simulink model "LICENTA_2024"  (R2018b)
settings: Solver=FixedStepDiscrete  StartTime=0.0  StopTime=Inf  RelTol=1e-3  EnableMultiTasking=on
values from neighbouring files (symbols this model uses):
  A = -Rs/Ld    (= -2.40983606557)    [licentam18.m]
  const_cuplu = 0.035    [licentam18.m]
  factor_conversie = (1/Rshunt)*(1/10)*(vref/4095)    (= 0.0115122972266)    [licentam18.m]
  FED = uint16(50)    [licentam18.m]
  MaxIter_1_ms_eCAP_wait = MinDetectSpeed_period/T_pos    (= 375)    [licentam18.m]
  pp = 16/2    (= 8)    [licentam18.m]
  RED = uint16(50)    [licentam18.m]
  T_pos = 0.0005    [licentam18.m]
  TBPRD1 = uint16(TPWM/(2*TTBCLK))    [licentam18.m]
  Tf = 0.015    [licentam18.m]
  Tf_spd = 0.01    [licentam18.m]
  Ts = Ts_crt_control    (= 3.33333333333e-05)    [licentam18.m]
  TTBCLK = 1/F    (= 5e-09)    [licentam18.m]
undefined symbols (not defined in the file or in its folder): Down, GPTRIP1SEL, GPTRIP2SEL, K, offset_ADC, radians, TZ1, TZ2, Up
libraries: tiiqmathlib x39, c2802xlib x9, c2837xDlib x6, simulink x5, c280xlib x4, c28xdmclib x2, c2000lib x1
(part 1 of 2)
settings Model: ExtModeTrigDuration=8  Creator=mocan  LastModifiedBy=mocan
settings SolverCC: AutoInsertRateTranBlk=on
settings OptimizationCC: DefaultUnderspecifiedDataType=single  EnhancedBackFolding=on  PassReuseOutputArgsAs=Individual arguments  MaxStackSize=512  OptimizeBlockOrder=speed  DifferentSizesBufferReuse=on  OptimizationCustomize=off
settings DebuggingCC: ParameterPrecisionLossMsg=none  ParameterTunabilityLossMsg=error
settings HardwareCC: ProdBitPerChar=16  ProdBitPerInt=16  ProdBitPerPointer=32  ProdBitPerSizeT=32  ProdBitPerPtrDiffT=32  ProdLargestAtomicInteger=Integer  ProdLargestAtomicFloat=None  ProdWordSize=16  ProdLongLongMode=on  ProdHWDeviceType=Texas Instruments->C2000
settings SFSimCC: MATLABDynamicMemAlloc=off
settings RTWCC: SystemTargetFile=ert.tlc  HardwareBoard=TI Delfino F28379D LaunchPad  TemplateMakefile=ert_default_tmf  GenerateReport=on  Toolchain=Texas Instruments Code Composer Studio (C2000)  IncludeHyperlinkInReport=on  LaunchReport=on  GenerateTraceInfo=on  GenerateTraceReport=on  GenerateTraceReportSl=on  GenerateTraceReportSf=on  GenerateTraceReportEml=on
settings CodeAppCC: ForceParamTrailComments=on  IgnoreCustomStorageClasses=off  OperatorAnnotations=on  SimulinkDataObjDesc=on  SFDataObjDesc=on  InsertBlockDesc=on
settings ERTTargetCC: CodeReplacementLibrary=TI C28x

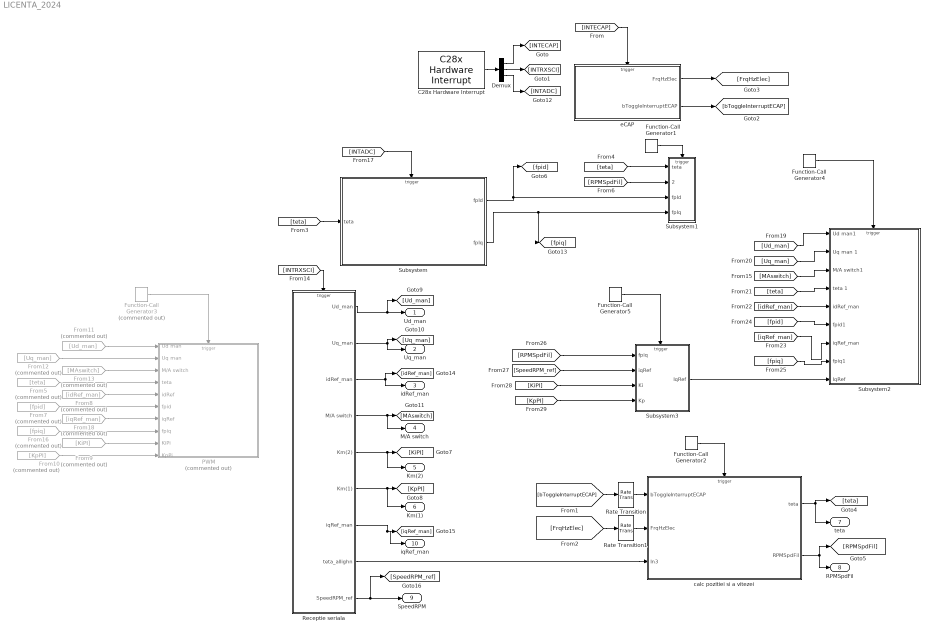
== system LICENTA_2024 ==
  C28x Hardware Interrupt : c2000lib/Scheduling/C28x Hardware Interrupt  irqnumbers=[4,9,1]  pienumbers=[1,1,1]  irqpriorities=[1, 1, 1]  irqpreempts=[0 0 0]  showinput=off  dspchiptype=C280X
      settings: SourceProductBaseCode=TIC2000
  Demux : Demux  Outputs=3
  From10 : From  Commented=on  GotoTag=KpPI
  From11 : From  Commented=on  GotoTag=Ud_man
  From12 : From  Commented=on  GotoTag=Uq_man
  From13 : From  Commented=on  GotoTag=MAswitch
  From16 : From  Commented=on  GotoTag=fpiq
  From18 : From  Commented=on  GotoTag=iqRef_man
  From5 : From  Commented=on  GotoTag=teta
  From7 : From  Commented=on  GotoTag=fpid
  From8 : From  Commented=on  GotoTag=idRef_man
  From9 : From  Commented=on  GotoTag=KiPI
  Function-Call Generator1 : simulink/Ports & Subsystems/Function-Call Generator  sample_time=0.03  numberOfIterations=1
  Function-Call Generator2 : simulink/Ports & Subsystems/Function-Call Generator  sample_time=T_pos  numberOfIterations=1
  Function-Call Generator3 : simulink/Ports & Subsystems/Function-Call Generator  Commented=on  sample_time=Ts_crt_control  numberOfIterations=1
  Function-Call Generator4 : simulink/Ports & Subsystems/Function-Call Generator  sample_time=Ts_crt_control  numberOfIterations=1
  Function-Call Generator5 : simulink/Ports & Subsystems/Function-Call Generator  sample_time=T_pos  numberOfIterations=1
  PWM : Subsystem  Commented=on
  Rate Transition : RateTransition  Integrity=off  OutPortSampleTime=T_pos
  Rate Transition1 : RateTransition  Integrity=off  OutPortSampleTime=T_pos
  "Receptie seriala " : Subsystem
  Subsystem : Subsystem
  Subsystem1 : Subsystem
  Subsystem2 : Subsystem
  Subsystem3 : Subsystem
  calc pozitiei si a vitezei : Subsystem
  eCAP : Subsystem
  Ud_man : Outport  VectorParamsAs1DForOutWhenUnconnected=on
  Uq_man : Outport  Port=2  VectorParamsAs1DForOutWhenUnconnected=on
  idRef_man : Outport  Port=3  VectorParamsAs1DForOutWhenUnconnected=on
  M/A switch : Outport  Port=4  VectorParamsAs1DForOutWhenUnconnected=on
  Km(2) : Outport  Port=5  VectorParamsAs1DForOutWhenUnconnected=on
  Km(1) : Outport  Port=6  VectorParamsAs1DForOutWhenUnconnected=on
  teta : Outport  Port=7  VectorParamsAs1DForOutWhenUnconnected=on
  RPMSpdFil : Outport  Port=8  VectorParamsAs1DForOutWhenUnconnected=on
  SpeedRPM : Outport  Port=9
  iqRef_man : Outport  Port=10
  wires:
  Rate Transition1/1 -> calc pozitiei si a vitezei/2(FrqHzElec)
  [FrqHzElec] -> Rate Transition1/1
  Rate Transition/1 -> calc pozitiei si a vitezei/1(bToggleInterruptECAP)
  [bToggleInterruptECAP] -> Rate Transition/1
  [INTECAP] -> eCAP/Trigger
  eCAP/1(FrqHzElec) -> [FrqHzElec]
  eCAP/2(bToggleInterruptECAP) -> [bToggleInterruptECAP]
  Demux/2 -> [INTRXSCI]
  Demux/1 -> [INTECAP]
  Function-Call Generator2/1 -> calc pozitiei si a vitezei/Trigger
  calc pozitiei si a vitezei/2(RPMSpdFil) -> [RPMSpdFil], RPMSpdFil/1
  Function-Call Generator1/1 -> Subsystem1/Trigger
  calc pozitiei si a vitezei/1(teta) -> [teta], teta/1
  [INTRXSCI] -> "Receptie seriala "/Trigger
  C28x Hardware Interrupt/1 -> Demux/1
  "Receptie seriala "/1(Ud_man) -> [Ud_man], Ud_man/1
  "Receptie seriala "/2(Uq_man) -> Uq_man/1, [Uq_man]
  "Receptie seriala "/4(M/A switch) -> M/A switch/1, [MAswitch]
  "Receptie seriala "/5(Km(2)) -> [KiPI], Km(2)/1
  "Receptie seriala "/6(Km(1)) -> Km(1)/1, [KpPI]
  Function-Call Generator3/1 -> PWM/Trigger
  Demux/3 -> [INTADC]
  [INTADC] -> Subsystem/Trigger
  [teta] -> Subsystem/1(teta)
  Subsystem/1(fpId) -> [fpid], Subsystem1/3(fpId)
  "Receptie seriala "/7(iqRef_man) -> iqRef_man/1, [iqRef_man]
  "Receptie seriala "/3(idRef_man) -> idRef_man/1, [idRef_man]
  From11/1 -> PWM/1(Ud man)
  From12/1 -> PWM/2("Uq man ")
  From13/1 -> PWM/3(M/A switch)
  From5/1 -> PWM/4("teta ")
  From8/1 -> PWM/5(idRef)
  From7/1 -> PWM/6(fpid)
  From16/1 -> PWM/8(fpiq)
  From18/1 -> PWM/7(iqRef)
  From9/1 -> PWM/9(KiPi)
  From10/1 -> PWM/10(KpPi)
  "Receptie seriala "/8(teta_allighn) -> calc pozitiei si a vitezei/3(In3)
  Function-Call Generator4/1 -> Subsystem2/Trigger
  [MAswitch] -> Subsystem2/3(M/A switch1)
  [Ud_man] -> Subsystem2/1(Ud man1)
  [teta] -> Subsystem2/4(teta 1)
  [idRef_man] -> Subsystem2/5(idRef_man)
  [iqRef_man] -> Subsystem2/7(iqRef_man)
  [fpid] -> Subsystem2/6(fpid1)
  [fpiq] -> Subsystem2/8(fpiq1)
  "Receptie seriala "/9(SpeedRPM_ref) -> SpeedRPM/1, [SpeedRPM_ref]
  [RPMSpdFil] -> Subsystem3/1(fpiq)
  [SpeedRPM_ref] -> Subsystem3/2(iqRef)
  Function-Call Generator5/1 -> Subsystem3/Trigger
  [Uq_man] -> Subsystem2/2(Uq man 1)
  Subsystem3/1(IqRef) -> Subsystem2/9(IqRef)
  Subsystem/2(fpIq) -> [fpiq], Subsystem1/4(fpIq)
  [teta] -> Subsystem1/1("teta ")
  [RPMSpdFil] -> Subsystem1/2("RPMSpdFil ")
  [KiPI] -> Subsystem3/3(Ki)
  [KpPI] -> Subsystem3/4(Kp)

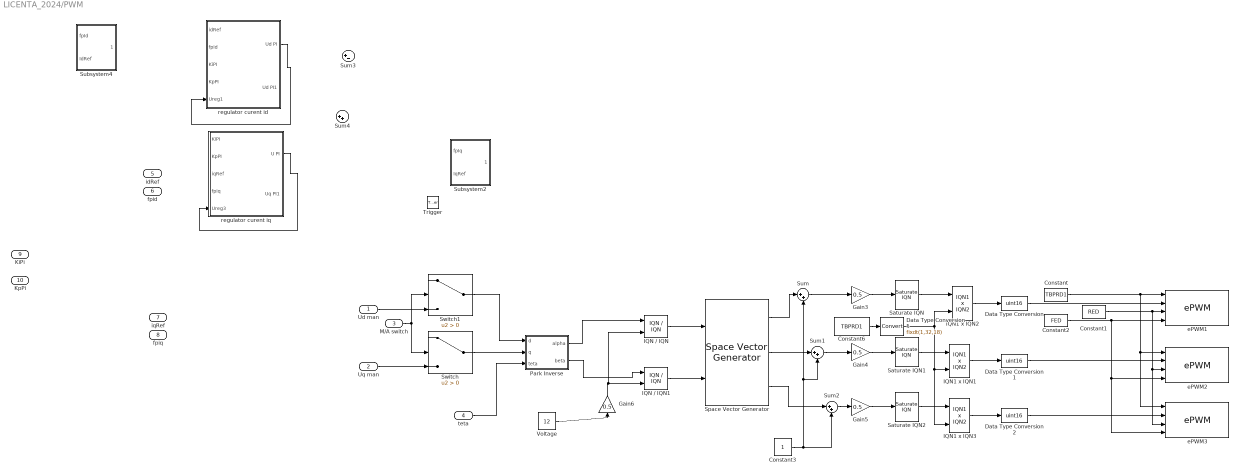
== system LICENTA_2024/PWM ==
  Ud man : Inport
  "Uq man " : Inport  Port=2
  M/A switch : Inport  Port=3
  "teta " : Inport  Port=4
  idRef : Inport  Port=5
  fpid : Inport  Port=6
  iqRef : Inport  Port=7
  fpiq : Inport  Port=8
  KiPi : Inport  Port=9
  KpPi : Inport  Port=10
  Trigger : TriggerPort  TriggerType=function-call  VariantControl=Variant  PortDimensions=1
  Constant : Constant  Value=TBPRD1
  Constant1 : Constant  Value=RED
  Constant2 : Constant  Value=FED
  Constant3 : Constant  OutDataTypeStr=fixdt(1,32,24)
  Constant6 : Constant  Value=TBPRD1
  Data Type Conversion : DataTypeConversion  OutDataTypeStr=uint16
  Data Type Conversion1 : DataTypeConversion  OutDataTypeStr=uint16
  Data Type Conversion2 : DataTypeConversion  OutDataTypeStr=uint16
  Data Type Conversion5 : DataTypeConversion  OutDataTypeStr=fixdt(1,32,18)
  Gain{3..6} (4 alike) : Gain  Gain=0.5  OutDataTypeStr=Inherit: Same as input
  IQN / IQN : tiiqmathlib/IQN // IQN
      settings: SourceProductName=Embedded Coder Support Package for Texas Instruments C2000 Processors  SourceProductBaseCode=TIC2000
  IQN / IQN1 : tiiqmathlib/IQN // IQN
      settings: SourceProductName=Embedded Coder Support Package for Texas Instruments C2000 Processors  SourceProductBaseCode=TIC2000
  IQN1 x IQN1 : tiiqmathlib/IQN1 x IQN2  Q=10
      settings: SourceProductName=Embedded Coder Support Package for Texas Instruments C2000 Processors  SourceProductBaseCode=TIC2000
  IQN1 x IQN2 : tiiqmathlib/IQN1 x IQN2  Q=10
      settings: SourceProductName=Embedded Coder Support Package for Texas Instruments C2000 Processors  SourceProductBaseCode=TIC2000
  IQN1 x IQN3 : tiiqmathlib/IQN1 x IQN2  Q=10
      settings: SourceProductName=Embedded Coder Support Package for Texas Instruments C2000 Processors  SourceProductBaseCode=TIC2000
  Park Inverse : Subsystem
  Saturate IQN : tiiqmathlib/Saturate IQN  pos=0.95  neg=0.05
      settings: SourceProductName=Embedded Coder Support Package for Texas Instruments C2000 Processors  SourceProductBaseCode=TIC2000
  Saturate IQN1 : tiiqmathlib/Saturate IQN  pos=0.95  neg=0.05
      settings: SourceProductName=Embedded Coder Support Package for Texas Instruments C2000 Processors  SourceProductBaseCode=TIC2000
  Saturate IQN2 : tiiqmathlib/Saturate IQN  pos=0.95  neg=0.05
      settings: SourceProductName=Embedded Coder Support Package for Texas Instruments C2000 Processors  SourceProductBaseCode=TIC2000
  Space Vector Generator : c28xdmclib/Space Vector Generator
      settings: SourceProductName=Embedded Coder Support Package for Texas Instruments C2000 Processors  SourceProductBaseCode=TIC2000
  Subsystem2 : Subsystem
  Subsystem4 : Subsystem
  Sum{,1..2,4} (4 alike) : Sum  Inputs=|++
  Sum3 : Sum  Inputs=|+-
  Switch : Switch  Criteria=u2 > Threshold
  Switch1 : Switch  Criteria=u2 > Threshold
  "Voltage " : Constant  Value=12  OutDataTypeStr=fixdt(1,32,20)
  ePWM1 : c2802xlib/ePWM  useModule=ePWM1  ePWMxLINKTBPRD=Not Linked  periodUnits=Clock cycles  timerSource=Input port  timerPeriod_clk=TBPRD1+1  timerPeriod_sec=0.0001  tbshadow=Counter equals to zero  countingMode=Up-Down  phaseActiveEnable=Disable  phaseDirection=Count up after sync  phaseActive=0  synchronizationEnable=off  dcaevt1Sync=off  dcbevt1Sync=off  synchronizationOption=Counter equals to zero (CTR=Zero)  clockPrescale=1  HSclockPrescale=1  enswap=off  ePWMxAStatus=on  ePWMxAactionLogic1=Do nothing  ePWMxAactionLogic2=Do nothing  ePWMxAactionLogic3=Clear  ePWMxAactionLogic4=Set  ePWMxAactionLogic5=Do nothing  ePWMxAactionLogic6=Do nothing  ePWMxALoadMode=Load on counter equals to zero (CTR=Zero)  ePWMxACSFenable=off  ePWMxACSFvalue=Forcing disable  ePWMxASFreload=Zero  ePWMxBStatus=off  ePWMxBactionLogic1=Set  ePWMxBactionLogic2=Clear  ePWMxBactionLogic3=Do nothing  ePWMxBactionLogic4=Do nothing  ePWMxBactionLogic5=Clear  ePWMxBactionLogic6=Set  ePWMxBLoadMode=Load on counter equals to zero (CTR=Zero)  ePWMxBCSFenable=off  ePWMxBCSFvalue=Forcing disable  ePWMxBSFreload=Zero  ePWNxBOutWay=off  ePWMxLINKCMPA=Not Linked  CMPAUnits=Clock cycles  CMPASource=Input port  CMPAValue_per=50  CMPAValue_clk=0  enCMPAshadow=Counter equals to zero  ePWMxLINKCMPB=Not Linked  CMPBUnits=Clock cycles  CMPBSource=Specify via dialog  CMPBValue_per=50  CMPBValue_clk=0  enCMPBshadow=Counter equals to zero  ePWMxLINKCMPC=Not Linked  CMPCUnits=Clock cycles  CMPCSource=Specify via dialog  CMPCValue_per=50  CMPCValue_clk=32000  enCMPCshadow=Counter equals to zero  ePWMxLINKCMPD=Not Linked  CMPDUnits=Clock cycles  CMPDSource=Specify via dialog  CMPDValue_per=50  CMPDValue_clk=32000  enCMPDshadow=Counter equals to zero  enableDBePWMxA=on  enableDBePWMxB=on  enhalfcycle=off  DBpolarity=Active high complementary (AHC)  DBedgeDelay=Positive  DBSource_ePWMxA=ePWMxA  DBSource_ePWMxB=ePWMxA  DBperiodSource=Input port  REDperiod=0  FEDperiod=0  adcstartModuleA=on  adcrequestEventA=First event  adcstartEventA=Digital Compare Module A Event 1 start of conversion (DCAEVT1.soc)  adcstartEventA_type2=Counter equals to period (CTR=PRD)  adcstartModuleB=off  adcrequestEventB=First event  adcstartEventB=Counter equals to zero (CTR=Zero)  adcstartEventB_type2=Counter equals to zero (CTR=Zero)  intEn=off  intPrd=First event  intSel=Counter equals to zero (CTR=Zero)  intSel_type2=Counter equals to zero (CTR=Zero)  hrpe=off  enHRPWM=off  HRPWM_LoadMode=Counter equals to period (CTR=PRD)  HRPWM_CTLMode=Duty or Period control mode  HRPWM_EDGMode=Both edge  hrpeb=off  enHRPWMB=off  HRPWM_LoadModeB=Counter equals to zero (CTR=ZERO)  HRPWM_CTLModeB=Duty or Period control mode  HRPWM_EDGModeB=Both edge  enSFO=on  enautoconv=on  chopperEnable=off  chopperFrequency=1  chopperFirstwidth=1  chopperDuty=12.5%  tripZonesource=Specify via dialog  tzselOSHT1=off  tzselOSHT2=off  tzselOSHT3=off  tzselOSHDCAEV1=off  tzselOSHDCBEV1=off  tzselCBC1=off  tzselCBC2=off  tzselCBC3=off  tzselCBCDCAEV2=off  tzselCBCDCBEV2=off  tzselOSHT4=off  tzselOSHT5=off  tzselOSHT6=off  tzselCBC4=off  tzselCBC5=off  tzselCBC6=off  enTzOstIntr=off  enTzCbcIntr=off  enTzDCAEVT1Intr=off  enTzDCAEVT2Intr=off  enTzDCBEVT1Intr=off  enTzDCBEVT2Intr=off  ePWMxAforced=No action  ePWMxBforced=No action  DCAEVT1forced=No action  DCBEVT1forced=No action  DCAEVT2forced=No action  DCBEVT2forced=No action  dcah=Trip Zone 1 input (TZ1)  dcal=Trip Zone 2 input (TZ2)  dcbh=Trip Zone 1 input (TZ1)  dcbl=Trip Zone 2 input (TZ2)  dcah_type2=GPTRIP1SEL/(TZ1)  dcal_type2=GPTRIP2SEL/(TZ2)  dcbh_type2=GPTRIP1SEL/(TZ1)  dcbl_type2=GPTRIP2SEL/(TZ2)  gendcaevt1=Event disabled  gendcaevt2=Event disabled  gendcbevt1=Event disabled  gendcbevt2=Event disabled  dcaevt1src=DCAEVT1 with sync  dcaevt2src=DCAEVT2 with sync  dcbevt1src=DCBEVT1 with sync  dcbevt2src=DCBEVT2 with sync  pulsesel=Counter equals to zero (CTR=Zero)  blankinv=off  blankoffset=0  blankwidth=0  evsrcsel=Filtered version of DCAEVT1 (DCAEVT1FILT)  encape=off  PwmType=C2000_Type4
      settings: SourceProductName=Embedded Coder Support Package for Texas Instruments C2000 Processors
  ePWM2 : c2802xlib/ePWM  useModule=ePWM2  ePWMxLINKTBPRD=Not Linked  periodUnits=Clock cycles  timerSource=Input port  timerPeriod_clk=TBPRD1+1  timerPeriod_sec=0.0001  tbshadow=Counter equals to zero  countingMode=Up-Down  phaseActiveEnable=Disable  phaseDirection=Count up after sync  phaseActive=0  synchronizationEnable=off  dcaevt1Sync=off  dcbevt1Sync=off  synchronizationOption=Counter equals to zero (CTR=Zero)  clockPrescale=1  HSclockPrescale=1  enswap=off  ePWMxAStatus=on  ePWMxAactionLogic1=Do nothing  ePWMxAactionLogic2=Do nothing  ePWMxAactionLogic3=Clear  ePWMxAactionLogic4=Set  ePWMxAactionLogic5=Do nothing  ePWMxAactionLogic6=Do nothing  ePWMxALoadMode=Load on counter equals to zero (CTR=Zero)  ePWMxACSFenable=off  ePWMxACSFvalue=Forcing disable  ePWMxASFreload=Zero  ePWMxBStatus=off  ePWMxBactionLogic1=Set  ePWMxBactionLogic2=Clear  ePWMxBactionLogic3=Do nothing  ePWMxBactionLogic4=Do nothing  ePWMxBactionLogic5=Clear  ePWMxBactionLogic6=Set  ePWMxBLoadMode=Load on counter equals to zero (CTR=Zero)  ePWMxBCSFenable=off  ePWMxBCSFvalue=Forcing disable  ePWMxBSFreload=Zero  ePWNxBOutWay=off  ePWMxLINKCMPA=Not Linked  CMPAUnits=Clock cycles  CMPASource=Input port  CMPAValue_per=50  CMPAValue_clk=0  enCMPAshadow=Counter equals to zero  ePWMxLINKCMPB=Not Linked  CMPBUnits=Clock cycles  CMPBSource=Specify via dialog  CMPBValue_per=50  CMPBValue_clk=0  enCMPBshadow=Counter equals to zero  ePWMxLINKCMPC=Not Linked  CMPCUnits=Clock cycles  CMPCSource=Specify via dialog  CMPCValue_per=50  CMPCValue_clk=32000  enCMPCshadow=Counter equals to zero  ePWMxLINKCMPD=Not Linked  CMPDUnits=Clock cycles  CMPDSource=Specify via dialog  CMPDValue_per=50  CMPDValue_clk=32000  enCMPDshadow=Counter equals to zero  enableDBePWMxA=on  enableDBePWMxB=on  enhalfcycle=off  DBpolarity=Active high complementary (AHC)  DBedgeDelay=Positive  DBSource_ePWMxA=ePWMxA  DBSource_ePWMxB=ePWMxA  DBperiodSource=Input port  REDperiod=0  FEDperiod=0  adcstartModuleA=on  adcrequestEventA=First event  adcstartEventA=Digital Compare Module A Event 1 start of conversion (DCAEVT1.soc)  adcstartEventA_type2=Counter equals to period (CTR=PRD)  adcstartModuleB=off  adcrequestEventB=First event  adcstartEventB=Counter equals to zero (CTR=Zero)  adcstartEventB_type2=Counter equals to zero (CTR=Zero)  intEn=off  intPrd=First event  intSel=Counter equals to zero (CTR=Zero)  intSel_type2=Counter equals to zero (CTR=Zero)  hrpe=off  enHRPWM=off  HRPWM_LoadMode=Counter equals to period (CTR=PRD)  HRPWM_CTLMode=Duty or Period control mode  HRPWM_EDGMode=Both edge  hrpeb=off  enHRPWMB=off  HRPWM_LoadModeB=Counter equals to zero (CTR=ZERO)  HRPWM_CTLModeB=Duty or Period control mode  HRPWM_EDGModeB=Both edge  enSFO=on  enautoconv=on  chopperEnable=off  chopperFrequency=1  chopperFirstwidth=1  chopperDuty=12.5%  tripZonesource=Specify via dialog  tzselOSHT1=off  tzselOSHT2=off  tzselOSHT3=off  tzselOSHDCAEV1=off  tzselOSHDCBEV1=off  tzselCBC1=off  tzselCBC2=off  tzselCBC3=off  tzselCBCDCAEV2=off  tzselCBCDCBEV2=off  tzselOSHT4=off  tzselOSHT5=off  tzselOSHT6=off  tzselCBC4=off  tzselCBC5=off  tzselCBC6=off  enTzOstIntr=off  enTzCbcIntr=off  enTzDCAEVT1Intr=off  enTzDCAEVT2Intr=off  enTzDCBEVT1Intr=off  enTzDCBEVT2Intr=off  ePWMxAforced=No action  ePWMxBforced=No action  DCAEVT1forced=No action  DCBEVT1forced=No action  DCAEVT2forced=No action  DCBEVT2forced=No action  dcah=Trip Zone 1 input (TZ1)  dcal=Trip Zone 2 input (TZ2)  dcbh=Trip Zone 1 input (TZ1)  dcbl=Trip Zone 2 input (TZ2)  dcah_type2=GPTRIP1SEL/(TZ1)  dcal_type2=GPTRIP2SEL/(TZ2)  dcbh_type2=GPTRIP1SEL/(TZ1)  dcbl_type2=GPTRIP2SEL/(TZ2)  gendcaevt1=Event disabled  gendcaevt2=Event disabled  gendcbevt1=Event disabled  gendcbevt2=Event disabled  dcaevt1src=DCAEVT1 with sync  dcaevt2src=DCAEVT2 with sync  dcbevt1src=DCBEVT1 with sync  dcbevt2src=DCBEVT2 with sync  pulsesel=Counter equals to zero (CTR=Zero)  blankinv=off  blankoffset=0  blankwidth=0  evsrcsel=Filtered version of DCAEVT1 (DCAEVT1FILT)  encape=off  PwmType=C2000_Type4
      settings: SourceProductName=Embedded Coder Support Package for Texas Instruments C2000 Processors
  ePWM3 : c2802xlib/ePWM  useModule=ePWM3  ePWMxLINKTBPRD=Not Linked  periodUnits=Clock cycles  timerSource=Input port  timerPeriod_clk=TBPRD1+1  timerPeriod_sec=0.0001  tbshadow=Counter equals to zero  countingMode=Up-Down  phaseActiveEnable=Disable  phaseDirection=Count up after sync  phaseActive=0  synchronizationEnable=off  dcaevt1Sync=off  dcbevt1Sync=off  synchronizationOption=Counter equals to zero (CTR=Zero)  clockPrescale=1  HSclockPrescale=1  enswap=off  ePWMxAStatus=on  ePWMxAactionLogic1=Do nothing  ePWMxAactionLogic2=Do nothing  ePWMxAactionLogic3=Clear  ePWMxAactionLogic4=Set  ePWMxAactionLogic5=Do nothing  ePWMxAactionLogic6=Do nothing  ePWMxALoadMode=Load on counter equals to zero (CTR=Zero)  ePWMxACSFenable=off  ePWMxACSFvalue=Forcing disable  ePWMxASFreload=Zero  ePWMxBStatus=off  ePWMxBactionLogic1=Set  ePWMxBactionLogic2=Clear  ePWMxBactionLogic3=Do nothing  ePWMxBactionLogic4=Do nothing  ePWMxBactionLogic5=Clear  ePWMxBactionLogic6=Set  ePWMxBLoadMode=Load on counter equals to zero (CTR=Zero)  ePWMxBCSFenable=off  ePWMxBCSFvalue=Forcing disable  ePWMxBSFreload=Zero  ePWNxBOutWay=off  ePWMxLINKCMPA=Not Linked  CMPAUnits=Clock cycles  CMPASource=Input port  CMPAValue_per=50  CMPAValue_clk=0  enCMPAshadow=Counter equals to zero  ePWMxLINKCMPB=Not Linked  CMPBUnits=Clock cycles  CMPBSource=Specify via dialog  CMPBValue_per=50  CMPBValue_clk=0  enCMPBshadow=Counter equals to zero  ePWMxLINKCMPC=Not Linked  CMPCUnits=Clock cycles  CMPCSource=Specify via dialog  CMPCValue_per=50  CMPCValue_clk=32000  enCMPCshadow=Counter equals to zero  ePWMxLINKCMPD=Not Linked  CMPDUnits=Clock cycles  CMPDSource=Specify via dialog  CMPDValue_per=50  CMPDValue_clk=32000  enCMPDshadow=Counter equals to zero  enableDBePWMxA=on  enableDBePWMxB=on  enhalfcycle=off  DBpolarity=Active high complementary (AHC)  DBedgeDelay=Positive  DBSource_ePWMxA=ePWMxA  DBSource_ePWMxB=ePWMxA  DBperiodSource=Input port  REDperiod=0  FEDperiod=0  adcstartModuleA=on  adcrequestEventA=First event  adcstartEventA=Digital Compare Module A Event 1 start of conversion (DCAEVT1.soc)  adcstartEventA_type2=Counter equals to period (CTR=PRD)  adcstartModuleB=off  adcrequestEventB=First event  adcstartEventB=Counter equals to zero (CTR=Zero)  adcstartEventB_type2=Counter equals to zero (CTR=Zero)  intEn=off  intPrd=First event  intSel=Counter equals to zero (CTR=Zero)  intSel_type2=Counter equals to zero (CTR=Zero)  hrpe=off  enHRPWM=off  HRPWM_LoadMode=Counter equals to period (CTR=PRD)  HRPWM_CTLMode=Duty or Period control mode  HRPWM_EDGMode=Both edge  hrpeb=off  enHRPWMB=off  HRPWM_LoadModeB=Counter equals to zero (CTR=ZERO)  HRPWM_CTLModeB=Duty or Period control mode  HRPWM_EDGModeB=Both edge  enSFO=on  enautoconv=on  chopperEnable=off  chopperFrequency=1  chopperFirstwidth=1  chopperDuty=12.5%  tripZonesource=Specify via dialog  tzselOSHT1=off  tzselOSHT2=off  tzselOSHT3=off  tzselOSHDCAEV1=off  tzselOSHDCBEV1=off  tzselCBC1=off  tzselCBC2=off  tzselCBC3=off  tzselCBCDCAEV2=off  tzselCBCDCBEV2=off  tzselOSHT4=off  tzselOSHT5=off  tzselOSHT6=off  tzselCBC4=off  tzselCBC5=off  tzselCBC6=off  enTzOstIntr=off  enTzCbcIntr=off  enTzDCAEVT1Intr=off  enTzDCAEVT2Intr=off  enTzDCBEVT1Intr=off  enTzDCBEVT2Intr=off  ePWMxAforced=No action  ePWMxBforced=No action  DCAEVT1forced=No action  DCBEVT1forced=No action  DCAEVT2forced=No action  DCBEVT2forced=No action  dcah=Trip Zone 1 input (TZ1)  dcal=Trip Zone 2 input (TZ2)  dcbh=Trip Zone 1 input (TZ1)  dcbl=Trip Zone 2 input (TZ2)  dcah_type2=GPTRIP1SEL/(TZ1)  dcal_type2=GPTRIP2SEL/(TZ2)  dcbh_type2=GPTRIP1SEL/(TZ1)  dcbl_type2=GPTRIP2SEL/(TZ2)  gendcaevt1=Event disabled  gendcaevt2=Event disabled  gendcbevt1=Event disabled  gendcbevt2=Event disabled  dcaevt1src=DCAEVT1 with sync  dcaevt2src=DCAEVT2 with sync  dcbevt1src=DCBEVT1 with sync  dcbevt2src=DCBEVT2 with sync  pulsesel=Counter equals to zero (CTR=Zero)  blankinv=off  blankoffset=0  blankwidth=0  evsrcsel=Filtered version of DCAEVT1 (DCAEVT1FILT)  encape=off  PwmType=C2000_Type4
      settings: SourceProductName=Embedded Coder Support Package for Texas Instruments C2000 Processors
  regulator curent id : Subsystem
  regulator curent iq : Subsystem
  wires:
  Constant/1 -> ePWM3/1, ePWM2/1, ePWM1/1
  Constant1/1 -> ePWM3/3, ePWM2/3, ePWM1/3
  Constant2/1 -> ePWM3/4, ePWM2/4, ePWM1/4
  Data Type Conversion/1 -> ePWM1/2
  Data Type Conversion1/1 -> ePWM2/2
  Data Type Conversion2/1 -> ePWM3/2
  IQN1 x IQN2/1 -> Data Type Conversion/1
  IQN1 x IQN1/1 -> Data Type Conversion1/1
  IQN1 x IQN3/1 -> Data Type Conversion2/1
  Saturate IQN/1 -> IQN1 x IQN2/1
  Saturate IQN1/1 -> IQN1 x IQN1/1
  Gain5/1 -> Saturate IQN2/1
  Gain4/1 -> Saturate IQN1/1
  Gain3/1 -> Saturate IQN/1
  Sum/1 -> Gain3/1
  Sum1/1 -> Gain4/1
  Sum2/1 -> Gain5/1
  Space Vector Generator/1 -> Sum/1
  Space Vector Generator/2 -> Sum1/1
  Space Vector Generator/3 -> Sum2/1
  Park Inverse/1(alpha) -> IQN / IQN/1
  Park Inverse/2(beta) -> IQN / IQN1/1
  Constant3/1 -> Sum1/2, Sum/2, Sum2/2
  "Voltage "/1 -> Gain6/1
  Gain6/1 -> IQN / IQN1/2, IQN / IQN/2
  M/A switch/1 -> Switch/2, Switch1/2
  "Uq man "/1 -> Switch/3
  "teta "/1 -> Park Inverse/3(teta)
  IQN / IQN/1 -> Space Vector Generator/1
  IQN / IQN1/1 -> Space Vector Generator/2
  Saturate IQN2/1 -> IQN1 x IQN3/1
  Switch/1 -> Park Inverse/2(q)
  Constant6/1 -> Data Type Conversion5/1
  Data Type Conversion5/1 -> IQN1 x IQN2/2, IQN1 x IQN3/2, IQN1 x IQN1/2
  Switch1/1 -> Park Inverse/1(d)
  Ud man/1 -> Switch1/3
  regulator curent id/1(Ud PI) -> regulator curent id/5(Ureg1)
  regulator curent iq/1(U PI) -> regulator curent iq/5(Ureg3)

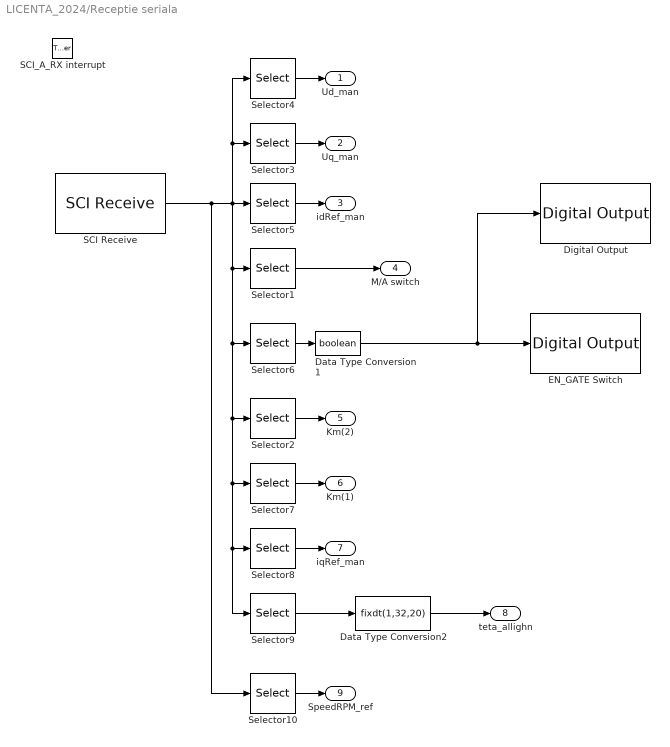
== system LICENTA_2024/Receptie seriala  ==
  "SCI_A_RX interrupt " : TriggerPort  TriggerType=function-call  VariantControl=(inherit)  PortDimensions=1
  Data Type Conversion1 : DataTypeConversion  OutDataTypeStr=boolean
  Data Type Conversion2 : DataTypeConversion  OutDataTypeStr=fixdt(1,32,20)
  Digital Output : c2837xDlib/Digital Output  GPIO_Number=GPIO88~GPIO95  GPIO_Bit0=off  GPIO_BIT0_Toggle=off  GPIO_Bit1=off  GPIO_BIT1_Toggle=off  GPIO_Bit2=off  GPIO_BIT2_Toggle=off  GPIO_Bit3=off  GPIO_BIT3_Toggle=off  GPIO_Bit4=off  GPIO_BIT4_Toggle=off  GPIO_Bit5=off  GPIO_BIT5_Toggle=off  GPIO_Bit6=on  GPIO_BIT6_Toggle=off  GPIO_Bit7=off  GPIO_BIT7_Toggle=off
      settings: SourceProductName=Embedded Coder Support Package for Texas Instruments C2000 Processors  SourceProductBaseCode=TIC2000
  EN_GATE Switch : c2837xDlib/Digital Output  GPIO_Number=GPIO120~GPIO127  GPIO_Bit0=off  GPIO_BIT0_Toggle=off  GPIO_Bit1=off  GPIO_BIT1_Toggle=off  GPIO_Bit2=off  GPIO_BIT2_Toggle=off  GPIO_Bit3=off  GPIO_BIT3_Toggle=off  GPIO_Bit4=on  GPIO_BIT4_Toggle=off  GPIO_Bit5=off  GPIO_BIT5_Toggle=off  GPIO_Bit6=off  GPIO_BIT6_Toggle=off  GPIO_Bit7=off  GPIO_BIT7_Toggle=on
      settings: SourceProductName=Embedded Coder Support Package for Texas Instruments C2000 Processors  SourceProductBaseCode=TIC2000
  SCI Receive : c280xlib/SCI Receive  sciModule=A  dataHead='SS'  dataTail='EE'  dataType=single  dataDim=serial_data_length  initValue=0  errOption=Output the last received value  errValue=0  sampleTime=-1  outputStatus=off  postInterrupt=on  numFifo=4
      settings: SourceProductName=Embedded Coder Support Package for Texas Instruments C2000 Processors  SourceProductBaseCode=TIC2000
  Selector1 : Selector  InputPortWidth=serial_data_length  IndexOptions=Index vector (dialog)  Indices=[4]  OutputSizes=1
  Selector10 : Selector  InputPortWidth=serial_data_length  IndexOptions=Index vector (dialog)  Indices=[10]  OutputSizes=1
  Selector2 : Selector  InputPortWidth=serial_data_length  IndexOptions=Index vector (dialog)  Indices=[6]  OutputSizes=1
  Selector3 : Selector  InputPortWidth=serial_data_length  IndexOptions=Index vector (dialog)  Indices=[2]  OutputSizes=1
  Selector4 : Selector  InputPortWidth=serial_data_length  IndexOptions=Index vector (dialog)  Indices=[1]  OutputSizes=1
  Selector5 : Selector  InputPortWidth=serial_data_length  IndexOptions=Index vector (dialog)  Indices=[3]  OutputSizes=1
  Selector6 : Selector  InputPortWidth=serial_data_length  IndexOptions=Index vector (dialog)  Indices=[5]  OutputSizes=1
  Selector7 : Selector  InputPortWidth=serial_data_length  IndexOptions=Index vector (dialog)  Indices=[7]  OutputSizes=1
  Selector8 : Selector  InputPortWidth=serial_data_length  IndexOptions=Index vector (dialog)  Indices=[8]  OutputSizes=1
  Selector9 : Selector  InputPortWidth=serial_data_length  IndexOptions=Index vector (dialog)  Indices=[9]  OutputSizes=1
  Ud_man : Outport  VectorParamsAs1DForOutWhenUnconnected=on
  Uq_man : Outport  Port=2  VectorParamsAs1DForOutWhenUnconnected=on
  idRef_man : Outport  Port=3  VectorParamsAs1DForOutWhenUnconnected=on
  M/A switch : Outport  Port=4  VectorParamsAs1DForOutWhenUnconnected=on
  Km(2) : Outport  Port=5  VectorParamsAs1DForOutWhenUnconnected=on
  Km(1) : Outport  Port=6  VectorParamsAs1DForOutWhenUnconnected=on
  iqRef_man : Outport  Port=7  VectorParamsAs1DForOutWhenUnconnected=on
  teta_allighn : Outport  Port=8  VectorParamsAs1DForOutWhenUnconnected=on
  SpeedRPM_ref : Outport  Port=9
  wires:
  SCI Receive/1 -> Selector10/1, Selector1/1, Selector6/1, Selector2/1, Selector9/1, Selector8/1, Selector7/1, Selector5/1, Selector4/1, Selector3/1
  Selector7/1 -> Km(1)/1
  Selector2/1 -> Km(2)/1
  Selector5/1 -> idRef_man/1
  Selector3/1 -> Uq_man/1
  Selector4/1 -> Ud_man/1
  Selector1/1 -> M/A switch/1
  Selector6/1 -> Data Type Conversion1/1
  Data Type Conversion1/1 -> Digital Output/1, EN_GATE Switch/1
  Selector8/1 -> iqRef_man/1
  Selector9/1 -> Data Type Conversion2/1
  Data Type Conversion2/1 -> teta_allighn/1
  Selector10/1 -> SpeedRPM_ref/1

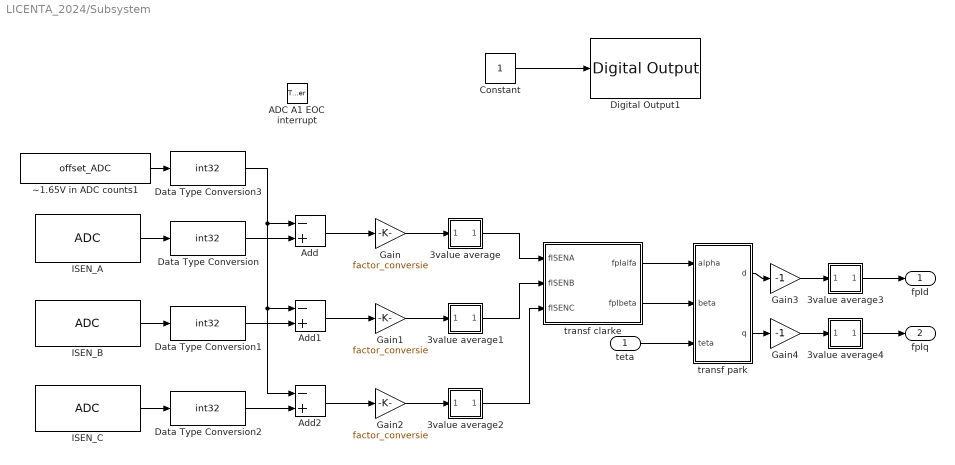
== system LICENTA_2024/Subsystem ==
  teta : Inport
  ADC A1 EOC interrupt : TriggerPort  TriggerType=function-call  VariantControl=Variant  PortDimensions=1
  3value average : Subsystem
  3value average1 : Subsystem
  3value average2 : Subsystem
  3value average3 : Subsystem
  3value average4 : Subsystem
  Add : Sum  Inputs=-+  OutDataTypeStr=single
  Add1 : Sum  Inputs=-+  OutDataTypeStr=single
  Add2 : Sum  Inputs=-+  OutDataTypeStr=single
  Constant : Constant
  Data Type Conversion{,1..3} (4 alike) : DataTypeConversion  OutDataTypeStr=int32  ConvertRealWorld=Stored Integer (SI)
  Digital Output1 : c2837xDlib/Digital Output  GPIO_Number=GPIO16~GPIO23  GPIO_Bit0=off  GPIO_BIT0_Toggle=off  GPIO_Bit1=off  GPIO_BIT1_Toggle=off  GPIO_Bit2=off  GPIO_BIT2_Toggle=off  GPIO_Bit3=off  GPIO_BIT3_Toggle=off  GPIO_Bit4=off  GPIO_BIT4_Toggle=off  GPIO_Bit5=off  GPIO_BIT5_Toggle=off  GPIO_Bit6=on  GPIO_BIT6_Toggle=on  GPIO_Bit7=off  GPIO_BIT7_Toggle=off
      settings: SourceProductName=Embedded Coder Support Package for Texas Instruments C2000 Processors  SourceProductBaseCode=TIC2000
  Gain : Gain  Gain=factor_conversie  OutDataTypeStr=fixdt(1,32,16)
  Gain1 : Gain  Gain=factor_conversie  OutDataTypeStr=fixdt(1,32,16)
  Gain2 : Gain  Gain=factor_conversie  OutDataTypeStr=fixdt(1,32,16)
  Gain3 : Gain  Gain=-1
  Gain4 : Gain  Gain=-1
  ISEN_A : c2802xlib/ADC  blkParamProc=C2000_Type4  ADCModule=C  samplingMode=Single sample mode  ADCResolution=12-bit (Single-ended input)  useSOC1=SOC0  useSOC2=SOC0_SOC1  SOCAcquisitionWindow=7  SOCTriggerSource=ePWM1_ADCSOCA  SOCInterruptTrigger=No ADCINT  Ts=-1  dType=uint16  postInterrupt=off  interruptSel=ADCINT2  ADCINTContinuous=on  endma=off  chdma=1  conv1=ADCINA0  conv2=ADCINA0 and ADCINB0  conv1_Type4=ADCIN2  conv2_Type4=ADCIN0 and ADCIN1
      settings: SourceProductName=Embedded Coder Support Package for Texas Instruments C2000 Processors
  ISEN_B : c2802xlib/ADC  blkParamProc=C2000_Type4  ADCModule=B  samplingMode=Single sample mode  ADCResolution=12-bit (Single-ended input)  useSOC1=SOC0  useSOC2=SOC0_SOC1  SOCAcquisitionWindow=7  SOCTriggerSource=ePWM1_ADCSOCA  SOCInterruptTrigger=No ADCINT  Ts=-1  dType=uint16  postInterrupt=off  interruptSel=ADCINT2  ADCINTContinuous=on  endma=off  chdma=1  conv1=ADCINA0  conv2=ADCINA0 and ADCINB0  conv1_Type4=ADCIN2  conv2_Type4=ADCIN0 and ADCIN1
      settings: SourceProductName=Embedded Coder Support Package for Texas Instruments C2000 Processors
  ISEN_C : c2802xlib/ADC  blkParamProc=C2000_Type4  ADCModule=A  samplingMode=Single sample mode  ADCResolution=12-bit (Single-ended input)  useSOC1=SOC0  useSOC2=SOC0_SOC1  SOCAcquisitionWindow=15  SOCTriggerSource=ePWM1_ADCSOCA  SOCInterruptTrigger=No ADCINT  Ts=-1  dType=uint16  postInterrupt=on  interruptSel=ADCINT1  ADCINTContinuous=on  endma=off  chdma=1  conv1=ADCINA0  conv2=ADCINA0 and ADCINB0  conv1_Type4=ADCIN2  conv2_Type4=ADCIN0 and ADCIN1
      settings: SourceProductName=Embedded Coder Support Package for Texas Instruments C2000 Processors
  transf clarke : Subsystem
  transf park : Subsystem
  ~1.65V in ADC counts1 : Constant  Value=offset_ADC  OutDataTypeStr=int32
  fpId : Outport
  fpIq : Outport  Port=2
  wires:
  3value average2/1(out) -> transf clarke/3(fISENC)
  3value average1/1(out) -> transf clarke/2(fISENB)
  3value average/1(out) -> transf clarke/1(fISENA)
  transf clarke/2(fpIbeta) -> transf park/2(beta)
  transf clarke/1(fpIalfa) -> transf park/1(alpha)
  teta/1 -> transf park/3("teta ")
  Data Type Conversion3/1 -> Add/1, Add1/1, Add2/1
  ISEN_B/1 -> Data Type Conversion1/1
  ISEN_C/1 -> Data Type Conversion2/1
  Data Type Conversion2/1 -> Add2/2
  Data Type Conversion1/1 -> Add1/2
  ~1.65V in ADC counts1/1 -> Data Type Conversion3/1
  Data Type Conversion/1 -> Add/2
  ISEN_A/1 -> Data Type Conversion/1
  Add/1 -> Gain/1
  Gain/1 -> 3value average/1(in)
  Add1/1 -> Gain1/1
  Gain1/1 -> 3value average1/1(in)
  Add2/1 -> Gain2/1
  Gain2/1 -> 3value average2/1(in)
  Constant/1 -> Digital Output1/1
  transf park/1(d) -> Gain3/1
  transf park/2(q) -> Gain4/1
  Gain3/1 -> 3value average3/1(in)
  Gain4/1 -> 3value average4/1(in)
  3value average3/1(out) -> fpId/1
  3value average4/1(out) -> fpIq/1

== system LICENTA_2024/Subsystem1 ==
  "teta " : Inport
  "RPMSpdFil " : Inport  Port=2
  fpId : Inport  Port=3
  fpIq : Inport  Port=4
  Trigger : TriggerPort  TriggerType=function-call  VariantControl=(inherit)  SampleTime=-1  PortDimensions=1
  Data Type Conversion{1..4} (4 alike) : DataTypeConversion  OutDataTypeStr=single
  Mux : Mux
  SCI Transmit : c280xlib/SCI Transmit  sciModule=A  dataHead='S'  dataTail='E'  postInterrupt=off  numFifo=1
      settings: SourceProductName=Embedded Coder Support Package for Texas Instruments C2000 Processors
  wires:
  "teta "/1 -> Data Type Conversion1/1
  "RPMSpdFil "/1 -> Data Type Conversion2/1
  Data Type Conversion2/1 -> Mux/2
  Mux/1 -> SCI Transmit/1
  Data Type Conversion1/1 -> Mux/1
  fpIq/1 -> Data Type Conversion4/1
  fpId/1 -> Data Type Conversion3/1
  Data Type Conversion3/1 -> Mux/3
  Data Type Conversion4/1 -> Mux/4
